simulink library "utility_service_lib"  (Simulink 8.1)
settings: Solver=ode45  StartTime=0.0  StopTime=10.0  RelTol=1e-3
undefined symbols (not defined in the file or in its folder): fdesignblkfcn, gcbh
libraries: rtio_opalrt_common x15, simulink x10, simulink_extras x8, rtio_opalrt_op5142ex1 x6, EasyGen3500_GensetSignalScaling_lib x2, rtlab x1
(part 1 of 2)
settings Model: Creator=RE25624  LastModifiedBy=RE25624

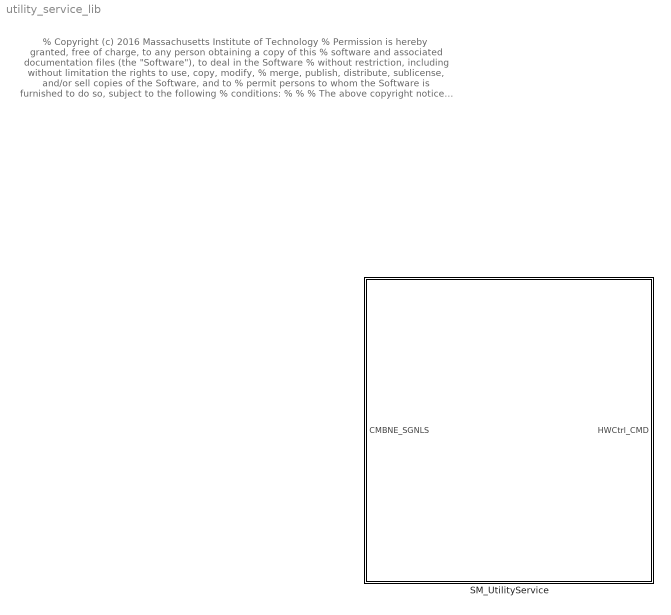
== system utility_service_lib ==
  note: % Copyright (c) 2016 Massachusetts Institute of Technology
      | % Permission is hereby granted, free of charge, to any person obtaining a copy of this
      | % software and associated documentation files (the "Software"), to deal in the Software
      | % without restriction, including without limitation the rights to use, copy, modify,
      | % merge, publish, distribute, sublicense, and/or sell copies of the Software, and to
      | % permit persons to whom the Software is furnished to do so, subject to the following
      | % conditions:
      | %
      | %
      | % The above copyright notice and this permission notice shall be included in
      | % all copies or substantial portions of the Software.
      | %
      | % THE SOFTWARE IS PROVIDED "AS IS", WITHOUT WARRANTY OF ANY KIND, EXPRESS OR IMPLIED,
      | % INCLUDING BUT NOT LIMITED TO THE WARRANTIES OF MERCHANTABILITY, FITNESS FOR A
      | % PARTICULAR PURPOSE AND NONINFRINGEMENT. IN NO EVENT SHALL THE AUTHORS OR COPYRIGHT
      | % HOLDERS BE LIABLE FOR ANY CLAIM, DAMAGES OR OTHER LIABILITY, WHETHER IN AN ACTION
      | % OF CONTRACT, TORT OR OTHERWISE, ARISING FROM, OUT OF OR IN CONNECTION WITH THE
      | % SOFTWARE OR THE USE OR OTHER DEALINGS IN THE SOFTWARE.
      | %
      | %
      | %%
  SM_UtilityService : Subsystem

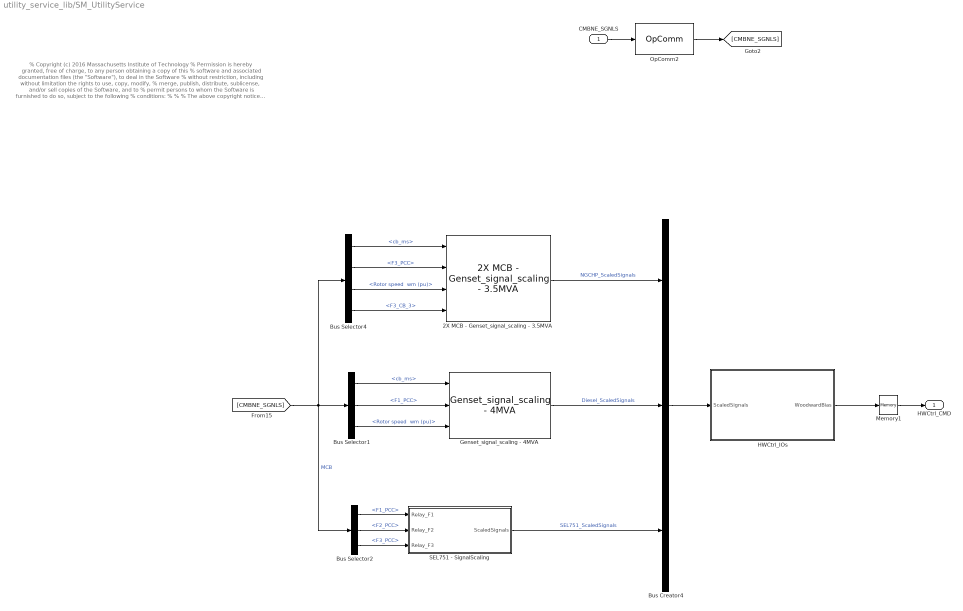
== system utility_service_lib/SM_UtilityService ==
  note: % Copyright (c) 2016 Massachusetts Institute of Technology
      | % Permission is hereby granted, free of charge, to any person obtaining a copy of this
      | % software and associated documentation files (the "Software"), to deal in the Software
      | % without restriction, including without limitation the rights to use, copy, modify,
      | % merge, publish, distribute, sublicense, and/or sell copies of the Software, and to
      | % permit persons to whom the Software is furnished to do so, subject to the following
      | % conditions:
      | %
      | %
      | % The above copyright notice and this permission notice shall be included in
      | % all copies or substantial portions of the Software.
      | %
      | % THE SOFTWARE IS PROVIDED "AS IS", WITHOUT WARRANTY OF ANY KIND, EXPRESS OR IMPLIED,
      | % INCLUDING BUT NOT LIMITED TO THE WARRANTIES OF MERCHANTABILITY, FITNESS FOR A
      | % PARTICULAR PURPOSE AND NONINFRINGEMENT. IN NO EVENT SHALL THE AUTHORS OR COPYRIGHT
      | % HOLDERS BE LIABLE FOR ANY CLAIM, DAMAGES OR OTHER LIABILITY, WHETHER IN AN ACTION
      | % OF CONTRACT, TORT OR OTHERWISE, ARISING FROM, OUT OF OR IN CONNECTION WITH THE
      | % SOFTWARE OR THE USE OR OTHER DEALINGS IN THE SOFTWARE.
      | %
      | %
      | %%
  CMBNE_SGNLS : Inport
  2X MCB - Genset_signal_scaling - 3.5MVA : EasyGen3500_GensetSignalScaling_lib/2X MCB - Genset_signal_scaling - 3.5MVA  Vpk_mcb=11268  watt_mcb=3150000  Vpk_gcb=11268  watt_gcb=3150000  rated_rpm=1800  wm_noise_bias=0.02
  Bus Creator4 : BusCreator  Inputs=3
  Bus Selector1 : BusSelector  OutputSignals="F1_MS_IN.DIESEL_DATA.DIESEL_GCB.cb_ms,F1_MS_IN.CB_DATA.F1_PCC,F1_MS_IN.DIESEL_DATA.Gen2_meas.w.w.Rotor speed  wm (pu)"
  Bus Selector2 : BusSelector  OutputSignals=F1_MS_IN.CB_DATA.F1_PCC,F2_MS_IN.CB_DATA.F2_PCC,F3_MS_IN.CB_DATA.F3_PCC
  Bus Selector4 : BusSelector  OutputSignals="F3_MS_IN.NG_CHP_DATA.NG_CHP_GCB.cb_ms,F3_MS_IN.CB_DATA.F3_PCC,F3_MS_IN.NG_CHP_DATA.Gen1_meas.w.w.Rotor speed  wm (pu),F3_MS_IN.CB_DATA.F3_CB_3"
  Genset_signal_scaling - 4MVA : EasyGen3500_GensetSignalScaling_lib/Genset_signal_scaling - 4MVA  Vpk_mcb=11268  watt_mcb=3600000  Vpk_gcb=11268  watt_gcb=3600000  rated_rpm=1800  wm_noise_bias=0.02
  HWCtrl_IOs : Subsystem
  Memory1 : Memory
  OpComm2 : rtlab/OpComm  nbport=1  groupe_acq=1  subsys_rate=0  st=0  Synchronization=on  Interpolation=on  Threshold=1.0  Missed_Data=off  Sim_Time=off  Samples=off  dynSigOut=off  from_console=0  warning_done=off  writeOpCommFile=off  Offset=off
  SEL751 - SignalScaling : Subsystem  mask(SEL751 - SignalScaling){ct_ratio=1/1250, pt_ratio=1/1800}
      mask prompts: ct_ratio "CT Ratio"; pt_ratio "PT Ratio"
      mask help: CT and PT ratios should match the settings in the corresponding SEL751
  HWCtrl_CMD : Outport
  wires:
  Bus Selector4/4 -> 2X MCB - Genset_signal_scaling - 3.5MVA/4  "<F3_CB_3>"
  Bus Selector2/3 -> SEL751 - SignalScaling/3(Relay_F3)  "<F3_PCC>"
  Bus Selector2/1 -> SEL751 - SignalScaling/1(Relay_F1)  "<F1_PCC>"
  Bus Selector2/2 -> SEL751 - SignalScaling/2(Relay_F2)  "<F2_PCC>"
  SEL751 - SignalScaling/1(ScaledSignals) -> Bus Creator4/3  "SEL751_ScaledSignals"
  OpComm2/1 -> [CMBNE_SGNLS]
  CMBNE_SGNLS/1 -> OpComm2/1
  Bus Selector1/1 -> Genset_signal_scaling - 4MVA/1  "<cb_ms>"
  Bus Selector1/2 -> Genset_signal_scaling - 4MVA/2  "<F1_PCC>"
  Bus Selector1/3 -> Genset_signal_scaling - 4MVA/3  "<Rotor speed  wm (pu)>"
  HWCtrl_IOs/1(WoodwardBias) -> Memory1/1
  Bus Creator4/1 -> HWCtrl_IOs/1(ScaledSignals)
  Bus Selector4/1 -> 2X MCB - Genset_signal_scaling - 3.5MVA/1  "<cb_ms>"
  Bus Selector4/2 -> 2X MCB - Genset_signal_scaling - 3.5MVA/2  "<F3_PCC>"
  Bus Selector4/3 -> 2X MCB - Genset_signal_scaling - 3.5MVA/3  "<Rotor speed  wm (pu)>"
  [CMBNE_SGNLS] -> Bus Selector1/1, Bus Selector2/1, Bus Selector4/1  "MCB"
  Genset_signal_scaling - 4MVA/1 -> Bus Creator4/2  "Diesel_ScaledSignals"
  2X MCB - Genset_signal_scaling - 3.5MVA/1 -> Bus Creator4/1  "NGCHP_ScaledSignals"
  Memory1/1 -> HWCtrl_CMD/1

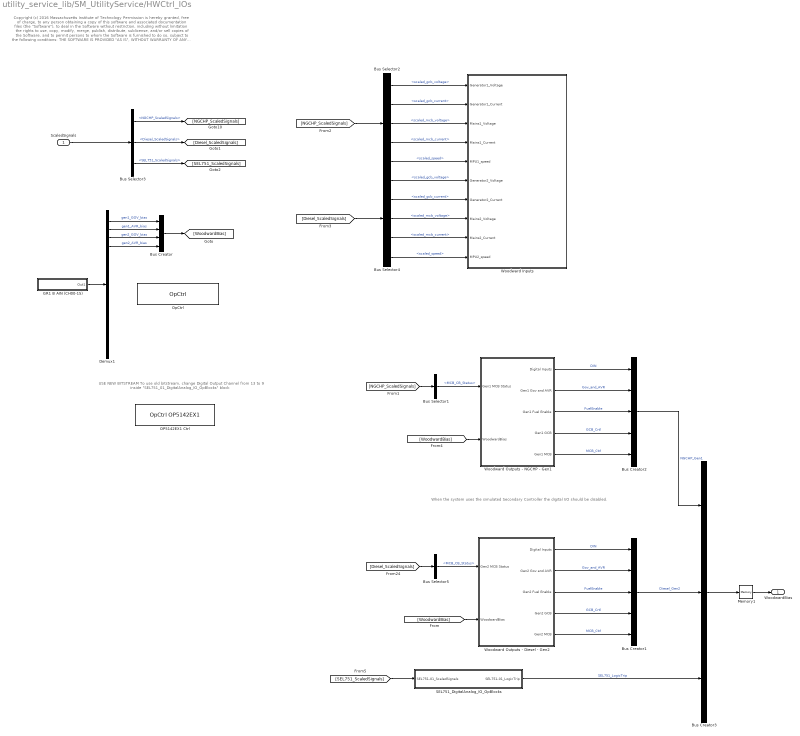
== system utility_service_lib/SM_UtilityService/HWCtrl_IOs ==
  note: USE NEW  BITSTREAM
      | To use old bitstream, change Digital Output Channel from 13 to 9 inside
      | "SEL751_01_DigitalAnalog_IO_OpBlocks" block
  note: Copyright (c) 2016 Massachusetts Institute of Technology
      | Permission is hereby granted, free of charge, to any person obtaining a copy of this software and associated documentation files (the "Software"), to deal
      | in the Software without restriction, including without limitation the rights to use, copy, modify, merge, publish, distribute, sublicense, and/or sell copies of the
      | Software, and to permit persons to whom the Software is furnished to do so, subject to the following conditions:
      |
      | THE SOFTWARE IS PROVIDED "AS IS", WITHOUT WARRANTY OF ANY KIND, EXPRESS OR IMPLIED, INCLUDING BUT NOT LIMITED TO THE
      | WARRANTIES OF MERCHANTABILITY, FITNESS FOR A PARTICULAR PURPOSE AND NONINFRINGEMENT. IN NO EVENT SHALL THE AUTHORS
      | OR COPYRIGHT HOLDERS BE LIABLE FOR ANY CLAIM, DAMAGES OR OTHER LIABILITY, WHETHER IN AN ACTION OF CONTRACT, TORT OR
      | OTHERWISE, ARISING FROM, OUT OF OR IN CONNECTION WITH THE SOFTWARE OR THE USE OR OTHER DEALINGS IN THE SOFTWARE
  note: When the system uses the simulated
      | Secondary Controller the digital I/O
      | should be disabled.
  ScaledSignals : Inport
  Bus Creator : BusCreator
  Bus Creator1 : BusCreator  Inputs=5
  Bus Creator2 : BusCreator  Inputs=5
  Bus Creator3 : BusCreator  Inputs=3
  Bus Selector1 : BusSelector  OutputSignals=MCB_CB_Status
  Bus Selector2 : BusSelector  OutputSignals=scaled_gcb_voltage,scaled_gcb_current,scaled_mcb_voltage,scaled_mcb_current,scaled_speed
  Bus Selector3 : BusSelector  OutputSignals=NGCHP_ScaledSignals,Diesel_ScaledSignals,SEL751_ScaledSignals
  Bus Selector4 : BusSelector  OutputSignals=scaled_gcb_voltage,scaled_gcb_current,scaled_mcb_voltage,scaled_mcb_current,scaled_speed
  Bus Selector5 : BusSelector  OutputSignals=MCB_CB_Status
  Demux1 : Demux  Outputs=16
  GR1 B AIN (CH00-15) : Subsystem
  Memory1 : Memory
  OP5142EX1 Ctrl : rtio_opalrt_op5142ex1/OpCtrl OP5142EX1  CtrlName='OP5142EX1 Ctrl'  boardid=1  BitstreamFilename=OP5142_1-EX-0000-2_3_4_54-16AIO_48AO_32DO_16DIO_16selDIO_CD-FF-01.bin  numconfig=-1  mode=Slave  externalClock=off  decimRtsi=0  calibIO=off  SampleTime=0  loadinport=-1
  OpCtrl : rtio_opalrt_common/OpCtrl  CtrlName='OpCtrl'  boardid=0  BitstreamFilename=VC707_2-EX-0001-2_3_2_20-48AIO16DIO16DIOSel-02-01.bin  numconfig=-1  mode=Master  externalClock=off  decimRtsi=0  calibIO=off  SampleTime=0  loadinport=-1  BoardType=VC707  SecondaryPresent=off  sync_type=Audio
  SEL751_DigitalAnalog_IO_OpBlocks : Subsystem
  Woodward Inputs : Subsystem
  Woodward Outputs - Diesel - Gen2 : Subsystem
  Woodward Outputs - NGCHP - Gen1 : Subsystem
  WoodwardBias : Outport
  wires:
  [SEL751_ScaledSignals] -> SEL751_DigitalAnalog_IO_OpBlocks/1(SEL751-01_ScaledSignals)
  Bus Selector3/3 -> [SEL751_ScaledSignals]  "<SEL751_ScaledSignals>"
  SEL751_DigitalAnalog_IO_OpBlocks/1(SEL751-01_LogicTrip) -> Bus Creator3/3  "SEL751_LogicTrip"
  ScaledSignals/1 -> Bus Selector3/1
  Bus Selector3/1 -> [NGCHP_ScaledSignals]  "<NGCHP_ScaledSignals>"
  Bus Selector3/2 -> [Diesel_ScaledSignals]  "<Diesel_ScaledSignals>"
  [NGCHP_ScaledSignals] -> Bus Selector2/1
  Bus Selector2/5 -> Woodward Inputs/5(MPU1_speed)  "<scaled_speed>"
  Bus Selector2/4 -> Woodward Inputs/4(Mains1_Current)  "<scaled_mcb_current>"
  Bus Selector2/3 -> Woodward Inputs/3(Mains1_Voltage)  "<scaled_mcb_voltage>"
  Bus Selector2/2 -> Woodward Inputs/2(Generator1_Current)  "<scaled_gcb_current>"
  Bus Selector2/1 -> Woodward Inputs/1(Generator1_Voltage)  "<scaled_gcb_voltage>"
  [Diesel_ScaledSignals] -> Bus Selector4/1
  Bus Selector4/1 -> Woodward Inputs/6(Generator2_Voltage)  "<scaled_gcb_voltage>"
  Bus Selector4/2 -> Woodward Inputs/7(Generator2_Current)  "<scaled_gcb_current>"
  Bus Selector4/3 -> Woodward Inputs/8(Mains2_Voltage)  "<scaled_mcb_voltage>"
  Bus Selector4/4 -> Woodward Inputs/9(Mains2_Current)  "<scaled_mcb_current>"
  Bus Selector4/5 -> Woodward Inputs/10(MPU2_speed)  "<scaled_speed>"
  GR1 B AIN (CH00-15)/1(Out1) -> Demux1/1
  Demux1/1 -> Bus Creator/1  "gen1_GOV_bias"
  Demux1/2 -> Bus Creator/2  "gen1_AVR_bias"
  Demux1/3 -> Bus Creator/3  "gen2_GOV_bias"
  Demux1/4 -> Bus Creator/4  "gen2_AVR_bias"
  Bus Selector5/1 -> Woodward Outputs - Diesel - Gen2/1(Gen2 MCB Status)  "<MCB_CB_Status>"
  [WoodwardBias] -> Woodward Outputs - Diesel - Gen2/2(WoodwardBias)
  [Diesel_ScaledSignals] -> Bus Selector5/1
  Woodward Outputs - Diesel - Gen2/2(Gen2 Gov and AVR) -> Bus Creator1/2  "Gov_and_AVR"
  Woodward Outputs - Diesel - Gen2/3(Gen2 Fuel Enable) -> Bus Creator1/3  "FuelEnable"
  Woodward Outputs - Diesel - Gen2/4(Gen2 GCB) -> Bus Creator1/4  "GCB_Crtl"
  Woodward Outputs - Diesel - Gen2/5(Gen2 MCB) -> Bus Creator1/5  "MCB_Ctrl"
  Bus Creator1/1 -> Bus Creator3/2  "Diesel_Gen2"
  Bus Creator3/1 -> Memory1/1
  Bus Creator2/1 -> Bus Creator3/1  "NGCHP_Gen1"
  Woodward Outputs - NGCHP - Gen1/1(Digital Inputs) -> Bus Creator2/1  "DIN"
  Woodward Outputs - NGCHP - Gen1/2(Gen1 Gov and AVR) -> Bus Creator2/2  "Gov_and_AVR"
  Woodward Outputs - NGCHP - Gen1/3(Gen1 Fuel Enable) -> Bus Creator2/3  "FuelEnable"
  Woodward Outputs - NGCHP - Gen1/4(Gen1 GCB) -> Bus Creator2/4  "GCB_Crtl"
  Woodward Outputs - Diesel - Gen2/1(Digital Inputs) -> Bus Creator1/1  "DIN"
  Woodward Outputs - NGCHP - Gen1/5(Gen1 MCB) -> Bus Creator2/5  "MCB_Ctrl"
  [WoodwardBias] -> Woodward Outputs - NGCHP - Gen1/2(WoodwardBias)
  [NGCHP_ScaledSignals] -> Bus Selector1/1
  Bus Selector1/1 -> Woodward Outputs - NGCHP - Gen1/1(Gen1 MCB Status)  "<MCB_CB_Status>"
  Memory1/1 -> WoodwardBias/1
  Bus Creator/1 -> [WoodwardBias]

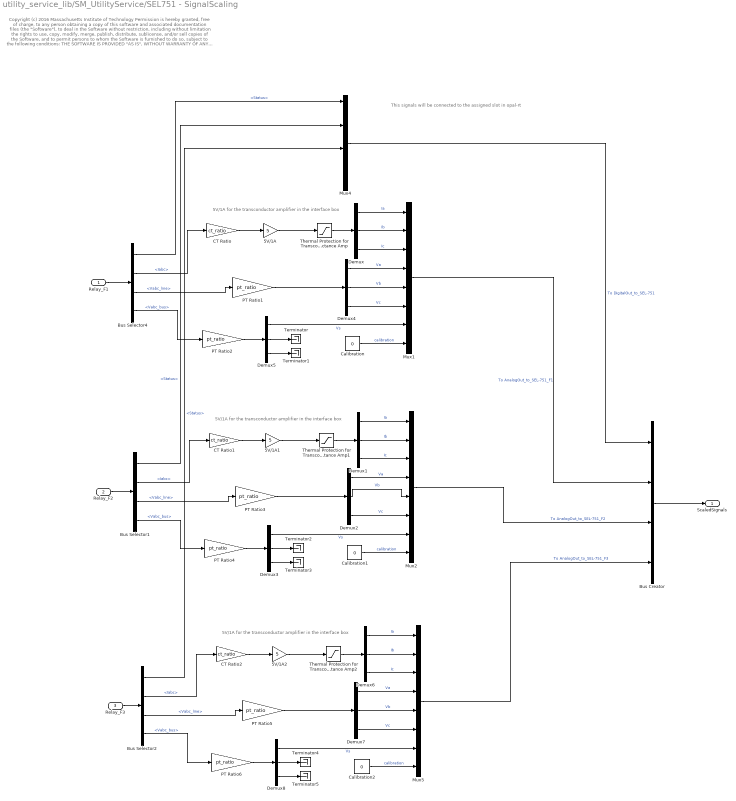
== system utility_service_lib/SM_UtilityService/SEL751 - SignalScaling ==
  note: Copyright (c) 2016 Massachusetts Institute of Technology
      | Permission is hereby granted, free of charge, to any person obtaining a copy of this software and associated documentation files (the "Software"), to deal
      | in the Software without restriction, including without limitation the rights to use, copy, modify, merge, publish, distribute, sublicense, and/or sell copies of the
      | Software, and to permit persons to whom the Software is furnished to do so, subject to the following conditions:
      |
      | THE SOFTWARE IS PROVIDED "AS IS", WITHOUT WARRANTY OF ANY KIND, EXPRESS OR IMPLIED, INCLUDING BUT NOT LIMITED TO THE
      | WARRANTIES OF MERCHANTABILITY, FITNESS FOR A PARTICULAR PURPOSE AND NONINFRINGEMENT. IN NO EVENT SHALL THE AUTHORS
      | OR COPYRIGHT HOLDERS BE LIABLE FOR ANY CLAIM, DAMAGES OR OTHER LIABILITY, WHETHER IN AN ACTION OF CONTRACT, TORT OR
      | OTHERWISE, ARISING FROM, OUT OF OR IN CONNECTION WITH THE SOFTWARE OR THE USE OR OTHER DEALINGS IN THE SOFTWARE
  note: This signals will be connected to the assigned slot in opal-rt
  note: 5V/1A for the transconductor
      | amplifier in the interface box
  note: 5V/1A for the transconductor
      | amplifier in the interface box
  note: 5V/1A for the transconductor
      | amplifier in the interface box
  Relay_F1 : Inport
  Relay_F2 : Inport  Port=2
  Relay_F3 : Inport  Port=3
  5V/1A : Gain  Gain=5
  5V/1A1 : Gain  Gain=5
  5V/1A2 : Gain  Gain=5
  Bus Creator : BusCreator
  Bus Selector1 : BusSelector  OutputSignals=Status,Iabc,Vabc_line,Vabc_bus
  Bus Selector2 : BusSelector  OutputSignals=Status,Iabc,Vabc_line,Vabc_bus
  Bus Selector4 : BusSelector  OutputSignals=Status,Iabc,Vabc_line,Vabc_bus
  CT Ratio : Gain  Gain=ct_ratio
  CT Ratio1 : Gain  Gain=ct_ratio
  CT Ratio2 : Gain  Gain=ct_ratio
  Calibration : Constant  Value=0
  Calibration1 : Constant  Value=0
  Calibration2 : Constant  Value=0
  Demux{,1..8} (9 alike) : Demux  Outputs=3
  Mux{1..2,4..5} (4 alike) : Mux  Inputs=8
  PT Ratio{1..6} (6 alike) : Gain  Gain=pt_ratio
  Terminator{,1..5} (6 alike) : Terminator
  Thermal Protection for Transconductance Amp : Saturate  UpperLimit=5  LowerLimit=-5
  Thermal Protection for Transconductance Amp1 : Saturate  UpperLimit=5  LowerLimit=-5
  Thermal Protection for Transconductance Amp2 : Saturate  UpperLimit=5  LowerLimit=-5
  ScaledSignals : Outport
  wires:
  5V/1A/1 -> Thermal Protection for Transconductance Amp/1
  Bus Creator/1 -> ScaledSignals/1
  Demux5/3 -> Terminator1/1
  Demux5/2 -> Terminator/1
  Thermal Protection for Transconductance Amp/1 -> Demux/1
  PT Ratio2/1 -> Demux5/1
  PT Ratio1/1 -> Demux4/1
  CT Ratio/1 -> 5V/1A/1
  Relay_F1/1 -> Bus Selector4/1
  Demux/2 -> Mux1/2  "Ib"
  Demux/3 -> Mux1/3  "Ic"
  Demux/1 -> Mux1/1  "Ia"
  Mux1/1 -> Bus Creator/2  "To AnalogOut_to_SEL-751_F1"
  Mux4/1 -> Bus Creator/1  "To DigitalOut_to_SEL-751"
  Bus Selector4/1 -> Mux4/1  "<Status>"
  Calibration/1 -> Mux1/8  "calibration"
  Bus Selector4/3 -> PT Ratio1/1  "<Vabc_line>"
  Demux5/1 -> Mux1/7  "Vs"
  Bus Selector4/4 -> PT Ratio2/1  "<Vabc_bus>"
  Demux4/3 -> Mux1/6  "Vc"
  Demux4/2 -> Mux1/5  "Vb"
  Demux4/1 -> Mux1/4  "Va"
  Bus Selector4/2 -> CT Ratio/1  "<Iabc>"
  5V/1A1/1 -> Thermal Protection for Transconductance Amp1/1
  Demux3/3 -> Terminator3/1
  Demux3/2 -> Terminator2/1
  Thermal Protection for Transconductance Amp1/1 -> Demux1/1
  PT Ratio4/1 -> Demux3/1
  PT Ratio3/1 -> Demux2/1
  CT Ratio1/1 -> 5V/1A1/1
  Demux1/2 -> Mux2/2  "Ib"
  Demux1/3 -> Mux2/3  "Ic"
  Demux1/1 -> Mux2/1  "Ia"
  Mux2/1 -> Bus Creator/3  "To AnalogOut_to_SEL-751_F2"
  Bus Selector1/1 -> Mux4/3  "<Status>"
  Calibration1/1 -> Mux2/8  "calibration"
  Bus Selector1/3 -> PT Ratio3/1  "<Vabc_line>"
  Demux3/1 -> Mux2/7  "Vs"
  Bus Selector1/4 -> PT Ratio4/1  "<Vabc_bus>"
  Demux2/3 -> Mux2/6  "Vc"
  Demux2/2 -> Mux2/5  "Vb"
  Demux2/1 -> Mux2/4  "Va"
  Bus Selector1/2 -> CT Ratio1/1  "<Iabc>"
  5V/1A2/1 -> Thermal Protection for Transconductance Amp2/1
  Demux8/3 -> Terminator5/1
  Demux8/2 -> Terminator4/1
  Thermal Protection for Transconductance Amp2/1 -> Demux6/1
  PT Ratio6/1 -> Demux8/1
  PT Ratio5/1 -> Demux7/1
  CT Ratio2/1 -> 5V/1A2/1
  Demux6/2 -> Mux5/2  "Ib"
  Demux6/3 -> Mux5/3  "Ic"
  Demux6/1 -> Mux5/1  "Ia"
  Mux5/1 -> Bus Creator/4  "To AnalogOut_to_SEL-751_F3"
  Bus Selector2/1 -> Mux4/5  "<Status>"
  Calibration2/1 -> Mux5/8  "calibration"
  Bus Selector2/3 -> PT Ratio5/1  "<Vabc_line>"
  Demux8/1 -> Mux5/7  "Vs"
  Bus Selector2/4 -> PT Ratio6/1  "<Vabc_bus>"
  Demux7/3 -> Mux5/6  "Vc"
  Demux7/2 -> Mux5/5  "Vb"
  Demux7/1 -> Mux5/4  "Va"
  Bus Selector2/2 -> CT Ratio2/1  "<Iabc>"
  Relay_F2/1 -> Bus Selector1/1
  Relay_F3/1 -> Bus Selector2/1

== system utility_service_lib/SM_UtilityService/HWCtrl_IOs/GR1 B AIN (CH00-15) ==
  AnalogIn : rtio_opalrt_common/AnalogIn  CtrlName='OpCtrl'  portNb=1  FcnNos=Slot 1 Module B Subsection 1  size=16  maxcount=8  count=8  numchan=8  sampleTime=0
      settings: AttributesFormatString=%<CtrlName>
  AnalogIn1 : rtio_opalrt_common/AnalogIn  CtrlName='OpCtrl'  portNb=2  FcnNos=Slot 1 Module B Subsection 2  size=16  maxcount=8  count=8  numchan=8  sampleTime=0
      settings: AttributesFormatString=%<CtrlName>
  Mux6 : Mux  Inputs=2
  Terminator2 : Terminator
  Terminator3 : Terminator
  Out1 : Outport
  wires:
  AnalogIn/1 -> Mux6/1
  AnalogIn1/1 -> Mux6/2
  AnalogIn/2 -> Terminator2/1
  AnalogIn1/2 -> Terminator3/1
  Mux6/1 -> Out1/1

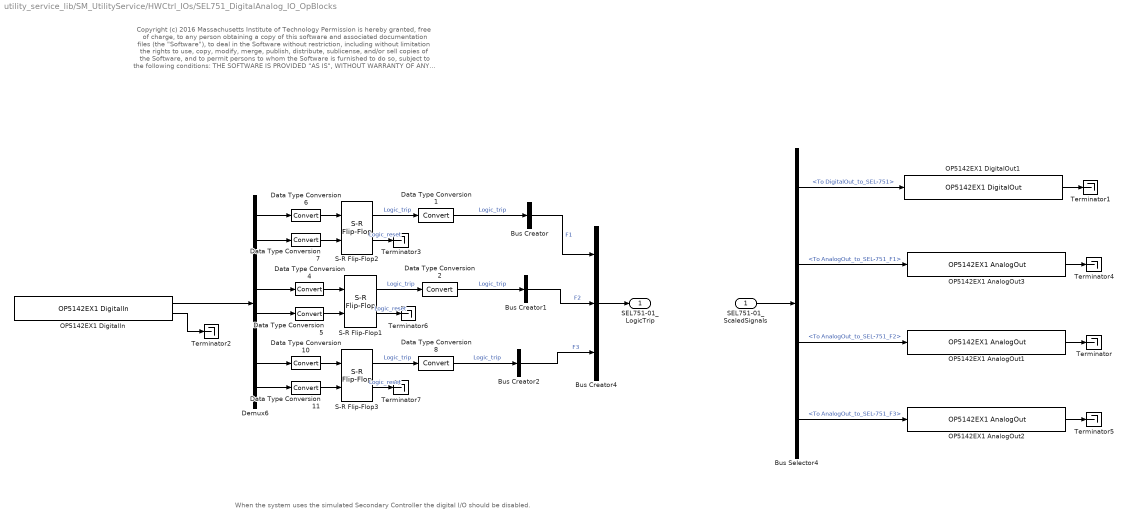
== system utility_service_lib/SM_UtilityService/HWCtrl_IOs/SEL751_DigitalAnalog_IO_OpBlocks ==
  note: Copyright (c) 2016 Massachusetts Institute of Technology
      | Permission is hereby granted, free of charge, to any person obtaining a copy of this software and associated documentation files (the "Software"), to deal
      | in the Software without restriction, including without limitation the rights to use, copy, modify, merge, publish, distribute, sublicense, and/or sell copies of the
      | Software, and to permit persons to whom the Software is furnished to do so, subject to the following conditions:
      |
      | THE SOFTWARE IS PROVIDED "AS IS", WITHOUT WARRANTY OF ANY KIND, EXPRESS OR IMPLIED, INCLUDING BUT NOT LIMITED TO THE
      | WARRANTIES OF MERCHANTABILITY, FITNESS FOR A PARTICULAR PURPOSE AND NONINFRINGEMENT. IN NO EVENT SHALL THE AUTHORS
      | OR COPYRIGHT HOLDERS BE LIABLE FOR ANY CLAIM, DAMAGES OR OTHER LIABILITY, WHETHER IN AN ACTION OF CONTRACT, TORT OR
      | OTHERWISE, ARISING FROM, OUT OF OR IN CONNECTION WITH THE SOFTWARE OR THE USE OR OTHER DEALINGS IN THE SOFTWARE
  note: When the system uses the simulated
      | Secondary Controller the digital I/O
      | should be disabled.
  SEL751-01_ScaledSignals : Inport
  Bus Creator : BusCreator  Inputs=1
  Bus Creator1 : BusCreator  Inputs=1
  Bus Creator2 : BusCreator  Inputs=1
  Bus Creator4 : BusCreator  Inputs=3
  Bus Selector4 : BusSelector  OutputSignals=To DigitalOut_to_SEL-751,To AnalogOut_to_SEL-751_F1,To AnalogOut_to_SEL-751_F2,To AnalogOut_to_SEL-751_F3
  Data Type Conversion{1..2,4..8,10..11} (9 alike) : DataTypeConversion
  Demux6 : Demux  Outputs=8
  OP5142EX1 AnalogOut1 : rtio_opalrt_op5142ex1/OP5142EX1 AnalogOut  CtrlName='OP5142EX1 Ctrl'  portNb=2  FcnNos=Slot 1 Module A Subsection 2  size=16  maxcount=8  count=8  numchan=8  israngeinput=off  voltagerange=[-16 ... 16]  slot=0  side=0  mismatch=0  slotside=Slot_1_Module_A
      settings: AttributesFormatString=%<CtrlName>
  OP5142EX1 AnalogOut2 : rtio_opalrt_op5142ex1/OP5142EX1 AnalogOut  CtrlName='OP5142EX1 Ctrl'  portNb=3  FcnNos=Slot 2 Module A Subsection 1  size=16  maxcount=8  count=8  numchan=8  israngeinput=off  voltagerange=[-16 ... 16]  slot=1  side=0  mismatch=0  slotside=Slot_2_Module_A
      settings: AttributesFormatString=%<CtrlName>
  OP5142EX1 AnalogOut3 : rtio_opalrt_op5142ex1/OP5142EX1 AnalogOut  CtrlName='OP5142EX1 Ctrl'  portNb=1  FcnNos=Slot 1 Module A Subsection 1  size=16  maxcount=8  count=8  numchan=8  israngeinput=off  voltagerange=[-16 ... 16]  slot=0  side=0  mismatch=0  slotside=Slot_1_Module_A
      settings: AttributesFormatString=%<CtrlName>
  OP5142EX1 DigitalIn : rtio_opalrt_op5142ex1/OP5142EX1 DigitalIn  CtrlName='OP5142EX1 Ctrl'  portNb=3  FcnNos=Slot 4 Module A Subsection 1  size=1  maxcount=8  count=8  sampleTime=0  numchan=8
      settings: AttributesFormatString=%<CtrlName>
  OP5142EX1 DigitalOut1 : rtio_opalrt_op5142ex1/OP5142EX1 DigitalOut  CtrlName='OP5142EX1 Ctrl'  portNb=13  FcnNos=Slot 4 Module B Subsection 1  size=1  maxcount=8  count=8  numchan=8
      settings: AttributesFormatString=%<CtrlName>
  S-R Flip-Flop1 : simulink_extras/Flip Flops/S-R Flip-Flop  initial_condition=1
  S-R Flip-Flop2 : simulink_extras/Flip Flops/S-R Flip-Flop  initial_condition=1
  S-R Flip-Flop3 : simulink_extras/Flip Flops/S-R Flip-Flop  initial_condition=1
  Terminator{,1..7} (8 alike) : Terminator
  SEL751-01_LogicTrip : Outport
  wires:
  Bus Selector4/2 -> OP5142EX1 AnalogOut3/1  "<To AnalogOut_to_SEL-751_F1>"
  Bus Selector4/3 -> OP5142EX1 AnalogOut1/1  "<To AnalogOut_to_SEL-751_F2>"
  Bus Selector4/4 -> OP5142EX1 AnalogOut2/1  "<To AnalogOut_to_SEL-751_F3>"
  S-R Flip-Flop2/2 -> Terminator3/1  "Logic_reset"
  S-R Flip-Flop1/2 -> Terminator6/1  "Logic_reset"
  S-R Flip-Flop3/2 -> Terminator7/1  "Logic_reset"
  Demux6/1 -> Data Type Conversion6/1
  Demux6/2 -> Data Type Conversion7/1
  Demux6/8 -> Data Type Conversion11/1
  Demux6/7 -> Data Type Conversion10/1
  S-R Flip-Flop3/1 -> Data Type Conversion8/1  "Logic_trip"
  Data Type Conversion10/1 -> S-R Flip-Flop3/1
  Data Type Conversion11/1 -> S-R Flip-Flop3/2
  S-R Flip-Flop2/1 -> Data Type Conversion1/1  "Logic_trip"
  Data Type Conversion6/1 -> S-R Flip-Flop2/1
  Data Type Conversion7/1 -> S-R Flip-Flop2/2
  S-R Flip-Flop1/1 -> Data Type Conversion2/1  "Logic_trip"
  OP5142EX1 DigitalIn/2 -> Terminator2/1
  OP5142EX1 DigitalIn/1 -> Demux6/1
  Data Type Conversion4/1 -> S-R Flip-Flop1/1
  Data Type Conversion5/1 -> S-R Flip-Flop1/2
  Demux6/4 -> Data Type Conversion4/1
  Demux6/5 -> Data Type Conversion5/1
  OP5142EX1 AnalogOut3/1 -> Terminator4/1
  OP5142EX1 AnalogOut2/1 -> Terminator5/1
  SEL751-01_ScaledSignals/1 -> Bus Selector4/1
  Bus Selector4/1 -> OP5142EX1 DigitalOut1/1  "<To DigitalOut_to_SEL-751>"
  OP5142EX1 AnalogOut1/1 -> Terminator/1
  OP5142EX1 DigitalOut1/1 -> Terminator1/1
  Bus Creator1/1 -> Bus Creator4/2  "F2"
  Bus Creator2/1 -> Bus Creator4/3  "F3"
  Bus Creator/1 -> Bus Creator4/1  "F1"
  Data Type Conversion8/1 -> Bus Creator2/1  "Logic_trip"
  Data Type Conversion2/1 -> Bus Creator1/1  "Logic_trip"
  Bus Creator4/1 -> SEL751-01_LogicTrip/1
  Data Type Conversion1/1 -> Bus Creator/1  "Logic_trip"

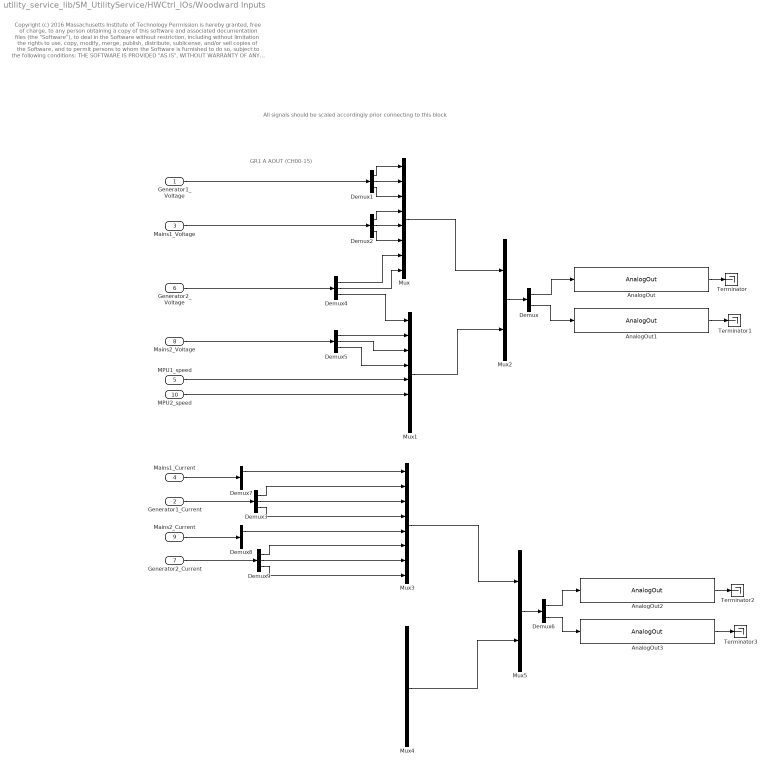
== system utility_service_lib/SM_UtilityService/HWCtrl_IOs/Woodward Inputs ==
  note: All signals should be scaled accordingly prior connecting to this block
  note: GR1 A AOUT (CH00-15)
  note: Copyright (c) 2016 Massachusetts Institute of Technology
      | Permission is hereby granted, free of charge, to any person obtaining a copy of this software and associated documentation files (the "Software"), to deal
      | in the Software without restriction, including without limitation the rights to use, copy, modify, merge, publish, distribute, sublicense, and/or sell copies of the
      | Software, and to permit persons to whom the Software is furnished to do so, subject to the following conditions:
      |
      | THE SOFTWARE IS PROVIDED "AS IS", WITHOUT WARRANTY OF ANY KIND, EXPRESS OR IMPLIED, INCLUDING BUT NOT LIMITED TO THE
      | WARRANTIES OF MERCHANTABILITY, FITNESS FOR A PARTICULAR PURPOSE AND NONINFRINGEMENT. IN NO EVENT SHALL THE AUTHORS
      | OR COPYRIGHT HOLDERS BE LIABLE FOR ANY CLAIM, DAMAGES OR OTHER LIABILITY, WHETHER IN AN ACTION OF CONTRACT, TORT OR
      | OTHERWISE, ARISING FROM, OUT OF OR IN CONNECTION WITH THE SOFTWARE OR THE USE OR OTHER DEALINGS IN THE SOFTWARE
  Generator1_Voltage : Inport
  Generator1_Current : Inport  Port=2
  Mains1_Voltage : Inport  Port=3
  Mains1_Current : Inport  Port=4
  MPU1_speed : Inport  Port=5
  Generator2_Voltage : Inport  Port=6
  Generator2_Current : Inport  Port=7
  Mains2_Voltage : Inport  Port=8
  Mains2_Current : Inport  Port=9
  MPU2_speed : Inport  Port=10
  AnalogOut : rtio_opalrt_common/AnalogOut  CtrlName='OpCtrl'  portNb=1  FcnNos=Slot 1 Module A Subsection 1  size=16  maxcount=8  count=8  numchan=8  israngeinput=off  voltagerange=[-16 ... 16]  slot=0  side=0  mismatch=0  slotside=Slot_1_Module_A
      settings: AttributesFormatString=%<CtrlName>
  AnalogOut1 : rtio_opalrt_common/AnalogOut  CtrlName='OpCtrl'  portNb=2  FcnNos=Slot 1 Module A Subsection 2  size=16  maxcount=8  count=8  numchan=8  israngeinput=off  voltagerange=[-16 ... 16]  slot=0  side=0  mismatch=0  slotside=Slot_1_Module_A
      settings: AttributesFormatString=%<CtrlName>
  AnalogOut2 : rtio_opalrt_common/AnalogOut  CtrlName='OpCtrl'  portNb=3  FcnNos=Slot 2 Module A Subsection 1  size=16  maxcount=8  count=8  numchan=8  israngeinput=off  voltagerange=[-16 ... 16]  slot=1  side=0  mismatch=0  slotside=Slot_2_Module_A
      settings: AttributesFormatString=%<CtrlName>
  AnalogOut3 : rtio_opalrt_common/AnalogOut  CtrlName='OpCtrl'  portNb=4  FcnNos=Slot 2 Module A Subsection 2  size=16  maxcount=8  count=8  numchan=8  israngeinput=off  voltagerange=[-16 ... 16]  slot=1  side=0  mismatch=0  slotside=Slot_2_Module_A
      settings: AttributesFormatString=%<CtrlName>
  Demux : Demux  Outputs=2
  Demux{1..5,7..9} (8 alike) : Demux  Outputs=3
  Demux6 : Demux  Outputs=2
  Mux{,1,3..4} (4 alike) : Mux  Inputs=8
  Mux2 : Mux  Inputs=2
  Mux5 : Mux  Inputs=2
  Terminator{,1..3} (4 alike) : Terminator
  wires:
  Demux9/3 -> Mux3/8
  Demux9/2 -> Mux3/7
  Demux9/1 -> Mux3/6
  Generator2_Current/1 -> Demux9/1
  Demux8/1 -> Mux3/5
  Mains2_Current/1 -> Demux8/1
  MPU2_speed/1 -> Mux1/6
  Generator2_Voltage/1 -> Demux4/1
  Mains2_Voltage/1 -> Demux5/1
  Demux7/1 -> Mux3/1
  Mains1_Current/1 -> Demux7/1
  Demux3/3 -> Mux3/4
  Demux3/2 -> Mux3/3
  Demux3/1 -> Mux3/2
  Generator1_Current/1 -> Demux3/1
  AnalogOut2/1 -> Terminator2/1
  AnalogOut3/1 -> Terminator3/1
  Demux6/1 -> AnalogOut2/1
  Demux6/2 -> AnalogOut3/1
  Mux3/1 -> Mux5/1
  Mux4/1 -> Mux5/2
  Mux5/1 -> Demux6/1
  Demux5/3 -> Mux1/4
  Demux5/2 -> Mux1/3
  Demux5/1 -> Mux1/2
  Demux4/3 -> Mux1/1
  Demux4/2 -> Mux/8
  Demux4/1 -> Mux/7
  MPU1_speed/1 -> Mux1/5
  Demux2/3 -> Mux/6
  Demux2/2 -> Mux/5
  Demux2/1 -> Mux/4
  Demux1/3 -> Mux/3
  Demux1/2 -> Mux/2
  Demux1/1 -> Mux/1
  AnalogOut/1 -> Terminator/1
  AnalogOut1/1 -> Terminator1/1
  Demux/1 -> AnalogOut/1
  Demux/2 -> AnalogOut1/1
  Mux/1 -> Mux2/1
  Mux1/1 -> Mux2/2
  Mux2/1 -> Demux/1
  Generator1_Voltage/1 -> Demux1/1
  Mains1_Voltage/1 -> Demux2/1

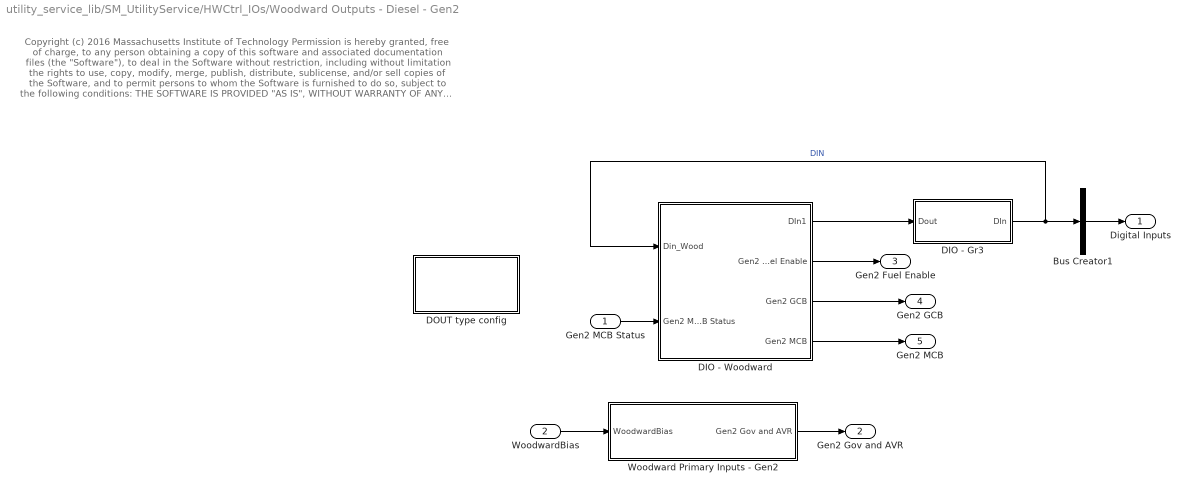
== system utility_service_lib/SM_UtilityService/HWCtrl_IOs/Woodward Outputs - Diesel - Gen2 ==
  note: Copyright (c) 2016 Massachusetts Institute of Technology
      | Permission is hereby granted, free of charge, to any person obtaining a copy of this software and associated documentation files (the "Software"), to deal
      | in the Software without restriction, including without limitation the rights to use, copy, modify, merge, publish, distribute, sublicense, and/or sell copies of the
      | Software, and to permit persons to whom the Software is furnished to do so, subject to the following conditions:
      |
      | THE SOFTWARE IS PROVIDED "AS IS", WITHOUT WARRANTY OF ANY KIND, EXPRESS OR IMPLIED, INCLUDING BUT NOT LIMITED TO THE
      | WARRANTIES OF MERCHANTABILITY, FITNESS FOR A PARTICULAR PURPOSE AND NONINFRINGEMENT. IN NO EVENT SHALL THE AUTHORS
      | OR COPYRIGHT HOLDERS BE LIABLE FOR ANY CLAIM, DAMAGES OR OTHER LIABILITY, WHETHER IN AN ACTION OF CONTRACT, TORT OR
      | OTHERWISE, ARISING FROM, OUT OF OR IN CONNECTION WITH THE SOFTWARE OR THE USE OR OTHER DEALINGS IN THE SOFTWARE
  Gen2 MCB Status : Inport
  WoodwardBias : Inport  Port=2
  Bus Creator1 : BusCreator  Inputs=1
  DIO - Gr3 : Subsystem
  DIO - Woodward : Subsystem
  DOUT type config : Subsystem
  Woodward Primary Inputs - Gen2 : Subsystem
  Digital Inputs : Outport
  Gen2 Gov and AVR : Outport  Port=2
  Gen2 Fuel Enable : Outport  Port=3
  Gen2 GCB : Outport  Port=4
  Gen2 MCB : Outport  Port=5
  wires:
  WoodwardBias/1 -> Woodward Primary Inputs - Gen2/1(WoodwardBias)
  Gen2 MCB Status/1 -> DIO - Woodward/2(Gen2 MCB Status)
  DIO - Woodward/4(Gen2 MCB) -> Gen2 MCB/1
  DIO - Woodward/2(Gen2 Fuel Enable) -> Gen2 Fuel Enable/1
  DIO - Woodward/3(Gen2 GCB) -> Gen2 GCB/1
  Woodward Primary Inputs - Gen2/1(Gen2 Gov and AVR) -> Gen2 Gov and AVR/1
  DIO - Gr3/1(DIn) -> DIO - Woodward/1(Din_Wood), Bus Creator1/1  "DIN"
  DIO - Woodward/1(DIn1) -> DIO - Gr3/1(Dout)
  Bus Creator1/1 -> Digital Inputs/1

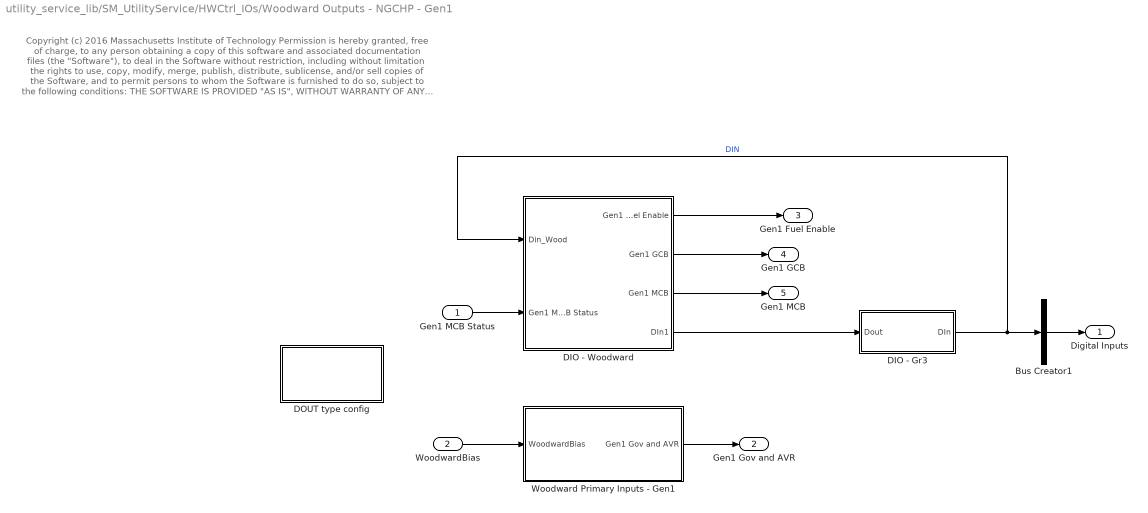
== system utility_service_lib/SM_UtilityService/HWCtrl_IOs/Woodward Outputs - NGCHP - Gen1 ==
  note: Copyright (c) 2016 Massachusetts Institute of Technology
      | Permission is hereby granted, free of charge, to any person obtaining a copy of this software and associated documentation files (the "Software"), to deal
      | in the Software without restriction, including without limitation the rights to use, copy, modify, merge, publish, distribute, sublicense, and/or sell copies of the
      | Software, and to permit persons to whom the Software is furnished to do so, subject to the following conditions:
      |
      | THE SOFTWARE IS PROVIDED "AS IS", WITHOUT WARRANTY OF ANY KIND, EXPRESS OR IMPLIED, INCLUDING BUT NOT LIMITED TO THE
      | WARRANTIES OF MERCHANTABILITY, FITNESS FOR A PARTICULAR PURPOSE AND NONINFRINGEMENT. IN NO EVENT SHALL THE AUTHORS
      | OR COPYRIGHT HOLDERS BE LIABLE FOR ANY CLAIM, DAMAGES OR OTHER LIABILITY, WHETHER IN AN ACTION OF CONTRACT, TORT OR
      | OTHERWISE, ARISING FROM, OUT OF OR IN CONNECTION WITH THE SOFTWARE OR THE USE OR OTHER DEALINGS IN THE SOFTWARE
  Gen1 MCB Status : Inport
  WoodwardBias : Inport  Port=2
  Bus Creator1 : BusCreator  Inputs=1
  DIO - Gr3 : Subsystem
  DIO - Woodward : Subsystem
  DOUT type config : Subsystem
  Woodward Primary Inputs - Gen1 : Subsystem
  Digital Inputs : Outport
  Gen1 Gov and AVR : Outport  Port=2
  Gen1 Fuel Enable : Outport  Port=3
  Gen1 GCB : Outport  Port=4
  Gen1 MCB : Outport  Port=5
  wires:
  Gen1 MCB Status/1 -> DIO - Woodward/2(Gen1 MCB Status)
  DIO - Woodward/1(Gen1 Fuel Enable) -> Gen1 Fuel Enable/1
  DIO - Woodward/3(Gen1 MCB) -> Gen1 MCB/1
  DIO - Woodward/2(Gen1 GCB) -> Gen1 GCB/1
  WoodwardBias/1 -> Woodward Primary Inputs - Gen1/1(WoodwardBias)
  Woodward Primary Inputs - Gen1/1(Gen1 Gov and AVR) -> Gen1 Gov and AVR/1
  Bus Creator1/1 -> Digital Inputs/1
  DIO - Gr3/1(DIn) -> Bus Creator1/1, DIO - Woodward/1(Din_Wood)  "DIN"
  DIO - Woodward/4(DIn1) -> DIO - Gr3/1(Dout)

== system utility_service_lib/SM_UtilityService/HWCtrl_IOs/Woodward Outputs - Diesel - Gen2/DIO - Gr3 ==
  Dout : Inport
  Bus Creator : BusCreator  Inputs=1
  Bus Selector1 : BusSelector  OutputSignals=DI_CH08-15  OutputAsBus=on
  Conditioning1 : Subsystem
  DigitalIn1 : rtio_opalrt_common/DigitalIn  CtrlName='OpCtrl'  portNb=6  FcnNos=Slot 3 Module A Subsection 2  size=1  maxcount=8  count=8  sampleTime=0  numchan=8
      settings: AttributesFormatString=%<CtrlName>
  DigitalOut1 : rtio_opalrt_common/DigitalOut  CtrlName='OpCtrl'  portNb=6  FcnNos=Slot 3 Module B Subsection 2  size=1  maxcount=8  count=8  numchan=8
      settings: AttributesFormatString=%<CtrlName>
  Terminator1 : Terminator
  Terminator6 : Terminator
  DIn : Outport
  wires:
  Conditioning1/1(Out1) -> Bus Creator/1
  Bus Creator/1 -> DIn/1
  DigitalIn1/1 -> Conditioning1/1(In1)  "DI_CH08-15"
  DigitalIn1/2 -> Terminator6/1
  Bus Selector1/1 -> DigitalOut1/1
  Dout/1 -> Bus Selector1/1
  DigitalOut1/1 -> Terminator1/1

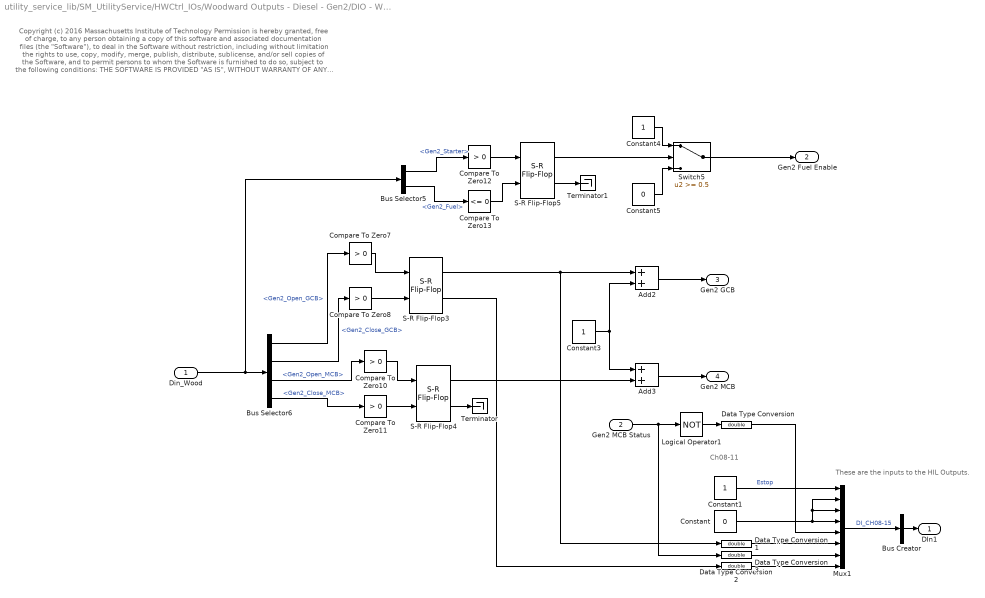
== system utility_service_lib/SM_UtilityService/HWCtrl_IOs/Woodward Outputs - Diesel - Gen2/DIO - Woodward ==
  note: These are the inputs to
      | the HIL Outputs.
  note: Ch08-11
  note: Copyright (c) 2016 Massachusetts Institute of Technology
      | Permission is hereby granted, free of charge, to any person obtaining a copy of this software and associated documentation files (the "Software"), to deal
      | in the Software without restriction, including without limitation the rights to use, copy, modify, merge, publish, distribute, sublicense, and/or sell copies of the
      | Software, and to permit persons to whom the Software is furnished to do so, subject to the following conditions:
      |
      | THE SOFTWARE IS PROVIDED "AS IS", WITHOUT WARRANTY OF ANY KIND, EXPRESS OR IMPLIED, INCLUDING BUT NOT LIMITED TO THE
      | WARRANTIES OF MERCHANTABILITY, FITNESS FOR A PARTICULAR PURPOSE AND NONINFRINGEMENT. IN NO EVENT SHALL THE AUTHORS
      | OR COPYRIGHT HOLDERS BE LIABLE FOR ANY CLAIM, DAMAGES OR OTHER LIABILITY, WHETHER IN AN ACTION OF CONTRACT, TORT OR
      | OTHERWISE, ARISING FROM, OUT OF OR IN CONNECTION WITH THE SOFTWARE OR THE USE OR OTHER DEALINGS IN THE SOFTWARE
  Din_Wood : Inport
  Gen2 MCB Status : Inport  Port=2
  Add2 : Sum
  Add3 : Sum
  Bus Creator : BusCreator  Inputs=1
  Bus Selector5 : BusSelector  OutputSignals=DI_CH08-15.Gen2_Starter,DI_CH08-15.Gen2_Fuel
  Bus Selector6 : BusSelector  OutputSignals=DI_CH08-15.Gen2_Open_GCB,DI_CH08-15.Gen2_Close_GCB,DI_CH08-15.Gen2_Open_MCB,DI_CH08-15.Gen2_Close_MCB
  Compare To Zero{7..8,10..12} (5 alike) : simulink/Logic and Bit Operations/Compare To Zero  relop=>  OutDataTypeStr=boolean
  Compare To Zero13 : simulink/Logic and Bit Operations/Compare To Zero  relop=<=  OutDataTypeStr=boolean
  Constant : Constant  Value=0
  Constant1 : Constant
  Constant3 : Constant
  Constant4 : Constant
  Constant5 : Constant  Value=0
  Data Type Conversion{,1..3} (4 alike) : DataTypeConversion  OutDataTypeStr=double
  Logical Operator1 : Logic  Operator=NOT  AllPortsSameDT=off  OutDataTypeStr=boolean
  Mux1 : Mux  Inputs=8
  S-R Flip-Flop3 : simulink_extras/Flip Flops/S-R Flip-Flop  initial_condition=1
  S-R Flip-Flop4 : simulink_extras/Flip Flops/S-R Flip-Flop  initial_condition=1
  S-R Flip-Flop5 : simulink_extras/Flip Flops/S-R Flip-Flop  initial_condition=0
  Switch5 : Switch  Threshold=0.5
  Terminator : Terminator
  Terminator1 : Terminator
  DIn1 : Outport
  Gen2 Fuel Enable : Outport  Port=2
  Gen2 GCB : Outport  Port=3
  Gen2 MCB : Outport  Port=4
  wires:
  Data Type Conversion/1 -> Mux1/5
  Logical Operator1/1 -> Data Type Conversion/1
  S-R Flip-Flop3/2 -> Data Type Conversion3/1
  Gen2 MCB Status/1 -> Data Type Conversion2/1, Logical Operator1/1
  Switch5/1 -> Gen2 Fuel Enable/1
  Compare To Zero13/1 -> S-R Flip-Flop5/2
  Constant4/1 -> Switch5/1
  Constant5/1 -> Switch5/3
  Compare To Zero12/1 -> S-R Flip-Flop5/1
  S-R Flip-Flop5/1 -> Switch5/2
  Bus Selector5/2 -> Compare To Zero13/1  "<Gen2_Fuel>"
  Bus Selector5/1 -> Compare To Zero12/1  "<Gen2_Starter>"
  Constant3/1 -> Add3/1, Add2/2
  Add3/1 -> Gen2 MCB/1
  Add2/1 -> Gen2 GCB/1
  S-R Flip-Flop4/1 -> Add3/2
  Bus Selector6/2 -> Compare To Zero8/1  "<Gen2_Close_GCB>"
  Compare To Zero10/1 -> S-R Flip-Flop4/1
  Bus Selector6/3 -> Compare To Zero10/1  "<Gen2_Open_MCB>"
  Compare To Zero11/1 -> S-R Flip-Flop4/2
  Bus Selector6/4 -> Compare To Zero11/1  "<Gen2_Close_MCB>"
  Compare To Zero8/1 -> S-R Flip-Flop3/2
  Compare To Zero7/1 -> S-R Flip-Flop3/1
  Bus Selector6/1 -> Compare To Zero7/1  "<Gen2_Open_GCB>"
  S-R Flip-Flop3/1 -> Add2/1, Data Type Conversion1/1
  Mux1/1 -> Bus Creator/1  "DI_CH08-15"
  Bus Creator/1 -> DIn1/1
  Din_Wood/1 -> Bus Selector6/1, Bus Selector5/1
  S-R Flip-Flop4/2 -> Terminator/1
  S-R Flip-Flop5/2 -> Terminator1/1
  Constant/1 -> Mux1/2, Mux1/3, Mux1/4
  Data Type Conversion1/1 -> Mux1/6
  Data Type Conversion2/1 -> Mux1/7
  Data Type Conversion3/1 -> Mux1/8
  Constant1/1 -> Mux1/1  "Estop"

== system utility_service_lib/SM_UtilityService/HWCtrl_IOs/Woodward Outputs - Diesel - Gen2/DOUT type config ==
  note: The Constants are used to select Digital Output type:
      | - 0: Time-Stamped Digital Output
      | - 1: Pulse-Width Modulated DIgital Output
  DataIn Send : rtio_opalrt_common/DataIn Send  CtrlName='OpCtrl'  FcnNos=11  width=1  portType=double  checkVersion=off  expectedId=0  expectedVersion=0  opComp=>=
      settings: AttributesFormatString=%<CtrlName>
  DataIn Send1 : rtio_opalrt_common/DataIn Send  CtrlName='OpCtrl'  FcnNos=12  width=1  portType=double  checkVersion=off  expectedId=0  expectedVersion=0  opComp=>=
      settings: AttributesFormatString=%<CtrlName>
  Subsection 3 DOUT type : Constant
  Subsection 4 DOUT type : Constant
  Terminator1 : Terminator
  Terminator2 : Terminator
  wires:
  DataIn Send/1 -> Terminator2/1
  DataIn Send1/1 -> Terminator1/1
  Subsection 4 DOUT type/1 -> DataIn Send1/1
  Subsection 3 DOUT type/1 -> DataIn Send/1

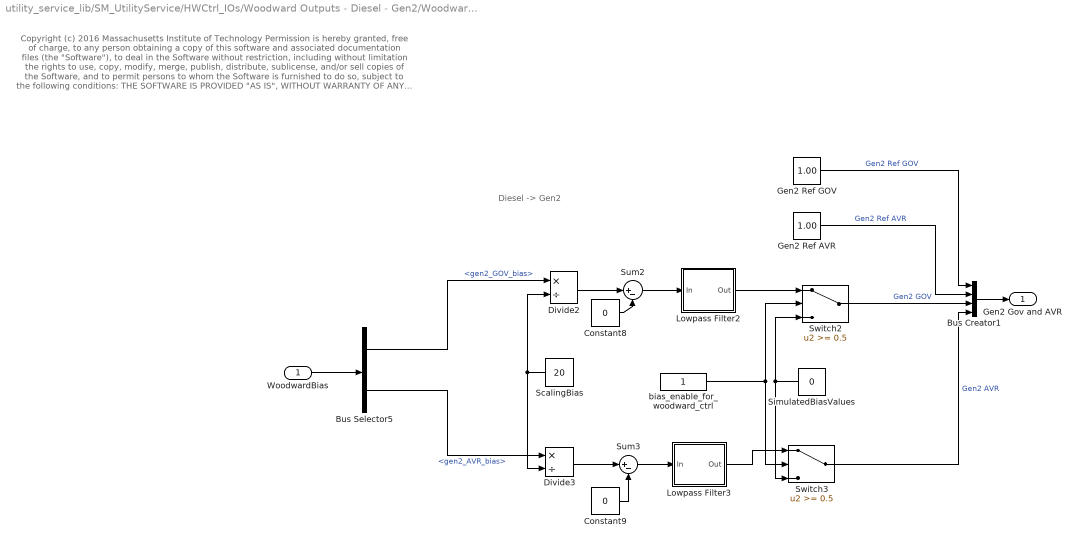
== system utility_service_lib/SM_UtilityService/HWCtrl_IOs/Woodward Outputs - Diesel - Gen2/Woodward Primary Inputs - Gen2 ==
  note: Diesel -> Gen2
  note: Copyright (c) 2016 Massachusetts Institute of Technology
      | Permission is hereby granted, free of charge, to any person obtaining a copy of this software and associated documentation files (the "Software"), to deal
      | in the Software without restriction, including without limitation the rights to use, copy, modify, merge, publish, distribute, sublicense, and/or sell copies of the
      | Software, and to permit persons to whom the Software is furnished to do so, subject to the following conditions:
      |
      | THE SOFTWARE IS PROVIDED "AS IS", WITHOUT WARRANTY OF ANY KIND, EXPRESS OR IMPLIED, INCLUDING BUT NOT LIMITED TO THE
      | WARRANTIES OF MERCHANTABILITY, FITNESS FOR A PARTICULAR PURPOSE AND NONINFRINGEMENT. IN NO EVENT SHALL THE AUTHORS
      | OR COPYRIGHT HOLDERS BE LIABLE FOR ANY CLAIM, DAMAGES OR OTHER LIABILITY, WHETHER IN AN ACTION OF CONTRACT, TORT OR
      | OTHERWISE, ARISING FROM, OUT OF OR IN CONNECTION WITH THE SOFTWARE OR THE USE OR OTHER DEALINGS IN THE SOFTWARE
  WoodwardBias : Inport
  Bus Creator1 : BusCreator
  Bus Selector5 : BusSelector  OutputSignals=gen2_GOV_bias,gen2_AVR_bias
  Constant8 : Constant  Value=0
  Constant9 : Constant  Value=0
  Divide2 : Product  Inputs=*/
  Divide3 : Product  Inputs=*/
  Gen2 Ref AVR : Constant  Value=1.00
  Gen2 Ref GOV : Constant  Value=1.00
  Lowpass Filter2 : Subsystem  DialogController=fdesignblkfcn  DialogControllerArgs=DataTag1  InitFcn=fdesignblkfcn(gcbh, {'InitFcn'});  mask(Lowpass Filter){}
      mask help: Design a lowpass filter
      settings: CopyFcn=fdesignblkfcn(gcbh, {'CopyFcn'});
      mask Help: helpview(mapfilelocation('dsp'), 'dsplowpassfilter');
      mask Display: disp('Lowpass')
  Lowpass Filter3 : Subsystem  DialogController=fdesignblkfcn  DialogControllerArgs=DataTag3  InitFcn=fdesignblkfcn(gcbh, {'InitFcn'});  mask(Lowpass Filter){}
      mask help: Design a lowpass filter
      settings: CopyFcn=fdesignblkfcn(gcbh, {'CopyFcn'});
      mask Help: helpview(mapfilelocation('dsp'), 'dsplowpassfilter');
      mask Display: disp('Lowpass')
  ScalingBias : Constant  Value=20
  SimulatedBiasValues : Constant  Value=0
  Sum2 : Sum  Inputs=|+-
  Sum3 : Sum  Inputs=|+-
  Switch2 : Switch  Threshold=0.5
  Switch3 : Switch  Threshold=0.5
  bias_enable_for_woodward_ctrl : Constant
  Gen2 Gov and AVR : Outport
  wires:
  Bus Selector5/2 -> Divide3/1  "<gen2_AVR_bias>"
  Bus Selector5/1 -> Divide2/1  "<gen2_GOV_bias>"
  WoodwardBias/1 -> Bus Selector5/1
  Bus Creator1/1 -> Gen2 Gov and AVR/1
  Gen2 Ref GOV/1 -> Bus Creator1/1  "Gen2 Ref GOV"
  Gen2 Ref AVR/1 -> Bus Creator1/2  "Gen2 Ref AVR"
  Lowpass Filter3/1(Out) -> Switch3/1
  Lowpass Filter2/1(Out) -> Switch2/1
  SimulatedBiasValues/1 -> Switch3/3, Switch2/3
  Sum3/1 -> Lowpass Filter3/1(In)
  Switch3/1 -> Bus Creator1/4  "Gen2 AVR"
  Switch2/1 -> Bus Creator1/3  "Gen2 GOV"
  Sum2/1 -> Lowpass Filter2/1(In)
  Constant9/1 -> Sum3/2
  Constant8/1 -> Sum2/2
  Divide3/1 -> Sum3/1
  Divide2/1 -> Sum2/1
  ScalingBias/1 -> Divide3/2, Divide2/2
  bias_enable_for_woodward_ctrl/1 -> Switch3/2, Switch2/2

== system utility_service_lib/SM_UtilityService/HWCtrl_IOs/Woodward Outputs - NGCHP - Gen1/DIO - Gr3 ==
  Dout : Inport
  Bus Creator : BusCreator  Inputs=1
  Bus Selector : BusSelector  OutputSignals=DI_CH00-07  OutputAsBus=on
  Conditioning : Subsystem
  DigitalIn : rtio_opalrt_common/DigitalIn  CtrlName='OpCtrl'  portNb=5  FcnNos=Slot 3 Module A Subsection 1  size=1  maxcount=8  count=8  sampleTime=0  numchan=8
      settings: AttributesFormatString=%<CtrlName>
  DigitalOut : rtio_opalrt_common/DigitalOut  CtrlName='OpCtrl'  portNb=5  FcnNos=Slot 3 Module B Subsection 1  size=1  maxcount=8  count=8  numchan=8
      settings: AttributesFormatString=%<CtrlName>
  Terminator3 : Terminator
  Terminator5 : Terminator
  DIn : Outport
  wires:
  Conditioning/1(Out1) -> Bus Creator/1
  Bus Creator/1 -> DIn/1
  DigitalIn/1 -> Conditioning/1(In1)  "DI_CH00-07"
  DigitalIn/2 -> Terminator5/1
  Bus Selector/1 -> DigitalOut/1
  Dout/1 -> Bus Selector/1
  DigitalOut/1 -> Terminator3/1

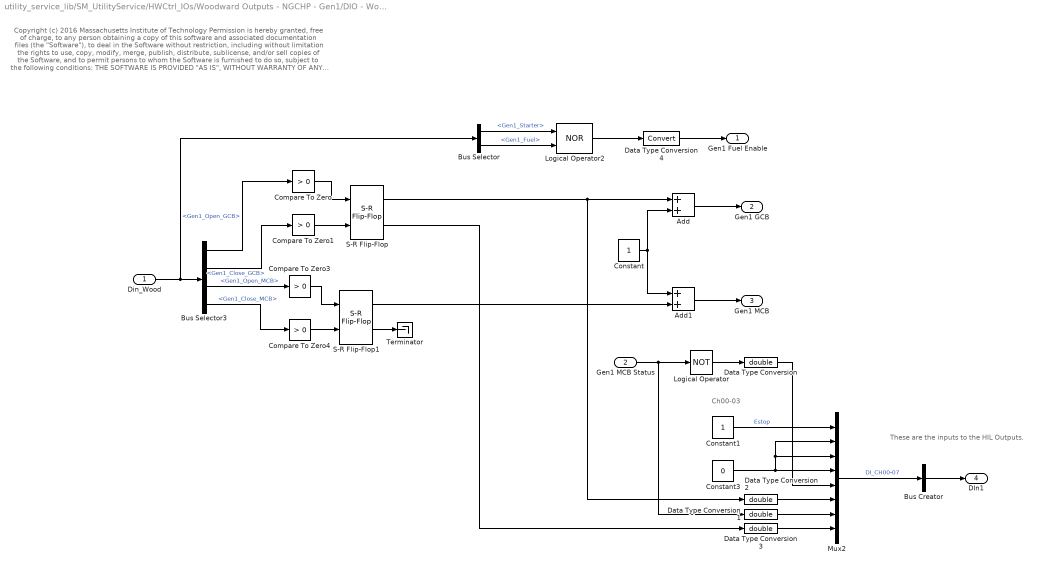
== system utility_service_lib/SM_UtilityService/HWCtrl_IOs/Woodward Outputs - NGCHP - Gen1/DIO - Woodward ==
  note: Copyright (c) 2016 Massachusetts Institute of Technology
      | Permission is hereby granted, free of charge, to any person obtaining a copy of this software and associated documentation files (the "Software"), to deal
      | in the Software without restriction, including without limitation the rights to use, copy, modify, merge, publish, distribute, sublicense, and/or sell copies of the
      | Software, and to permit persons to whom the Software is furnished to do so, subject to the following conditions:
      |
      | THE SOFTWARE IS PROVIDED "AS IS", WITHOUT WARRANTY OF ANY KIND, EXPRESS OR IMPLIED, INCLUDING BUT NOT LIMITED TO THE
      | WARRANTIES OF MERCHANTABILITY, FITNESS FOR A PARTICULAR PURPOSE AND NONINFRINGEMENT. IN NO EVENT SHALL THE AUTHORS
      | OR COPYRIGHT HOLDERS BE LIABLE FOR ANY CLAIM, DAMAGES OR OTHER LIABILITY, WHETHER IN AN ACTION OF CONTRACT, TORT OR
      | OTHERWISE, ARISING FROM, OUT OF OR IN CONNECTION WITH THE SOFTWARE OR THE USE OR OTHER DEALINGS IN THE SOFTWARE
  note: Ch00-03
  note: These are the inputs to
      | the HIL Outputs.
  Din_Wood : Inport
  Gen1 MCB Status : Inport  Port=2
  Add : Sum
  Add1 : Sum
  Bus Creator : BusCreator  Inputs=1
  Bus Selector : BusSelector  OutputSignals=DI_CH00-07.Gen1_Starter,DI_CH00-07.Gen1_Fuel
  Bus Selector3 : BusSelector  OutputSignals=DI_CH00-07.Gen1_Open_GCB,DI_CH00-07.Gen1_Close_GCB,DI_CH00-07.Gen1_Open_MCB,DI_CH00-07.Gen1_Close_MCB
  Compare To Zero{,1,3..4} (4 alike) : simulink/Logic and Bit Operations/Compare To Zero  relop=>  OutDataTypeStr=boolean
  Constant : Constant
  Constant1 : Constant
  Constant3 : Constant  Value=0
  Data Type Conversion{,1..3} (4 alike) : DataTypeConversion  OutDataTypeStr=double
  Data Type Conversion4 : DataTypeConversion
  Logical Operator : Logic  Operator=NOT  AllPortsSameDT=off  OutDataTypeStr=boolean
  Logical Operator2 : Logic  Operator=NOR  AllPortsSameDT=off  OutDataTypeStr=boolean
  Mux2 : Mux  Inputs=8
  S-R Flip-Flop : simulink_extras/Flip Flops/S-R Flip-Flop  initial_condition=1
  S-R Flip-Flop1 : simulink_extras/Flip Flops/S-R Flip-Flop  initial_condition=1
  Terminator : Terminator
  Gen1 Fuel Enable : Outport
  Gen1 GCB : Outport  Port=2
  Gen1 MCB : Outport  Port=3
  DIn1 : Outport  Port=4
  wires:
  S-R Flip-Flop1/2 -> Terminator/1
  Data Type Conversion2/1 -> Mux2/6
  Data Type Conversion1/1 -> Mux2/7
  Data Type Conversion3/1 -> Mux2/8
  Mux2/1 -> Bus Creator/1  "DI_CH00-07"
  Constant3/1 -> Mux2/2, Mux2/3, Mux2/4
  Logical Operator2/1 -> Data Type Conversion4/1
  Logical Operator/1 -> Data Type Conversion/1
  Data Type Conversion/1 -> Mux2/5
  S-R Flip-Flop/2 -> Data Type Conversion3/1
  Gen1 MCB Status/1 -> Logical Operator/1, Data Type Conversion1/1
  Bus Selector3/3 -> Compare To Zero3/1  "<Gen1_Open_MCB>"
  Bus Selector/2 -> Logical Operator2/2  "<Gen1_Fuel>"
  Bus Selector/1 -> Logical Operator2/1  "<Gen1_Starter>"
  Constant/1 -> Add1/1, Add/2
  Add1/1 -> Gen1 MCB/1
  Add/1 -> Gen1 GCB/1
  S-R Flip-Flop1/1 -> Add1/2
  Compare To Zero3/1 -> S-R Flip-Flop1/1
  Compare To Zero4/1 -> S-R Flip-Flop1/2
  Bus Selector3/4 -> Compare To Zero4/1  "<Gen1_Close_MCB>"
  Compare To Zero1/1 -> S-R Flip-Flop/2
  Compare To Zero/1 -> S-R Flip-Flop/1
  S-R Flip-Flop/1 -> Data Type Conversion2/1, Add/1
  Bus Creator/1 -> DIn1/1
  Din_Wood/1 -> Bus Selector/1, Bus Selector3/1
  Bus Selector3/1 -> Compare To Zero/1  "<Gen1_Open_GCB>"
  Bus Selector3/2 -> Compare To Zero1/1  "<Gen1_Close_GCB>"
  Data Type Conversion4/1 -> Gen1 Fuel Enable/1
  Constant1/1 -> Mux2/1  "Estop"

== system utility_service_lib/SM_UtilityService/HWCtrl_IOs/Woodward Outputs - NGCHP - Gen1/DOUT type config ==
  note: The Constants are used to select Digital Output type:
      | - 0: Time-Stamped Digital Output
      | - 1: Pulse-Width Modulated DIgital Output
  DataIn Send : rtio_opalrt_common/DataIn Send  CtrlName='OpCtrl'  FcnNos=11  width=1  portType=double  checkVersion=off  expectedId=0  expectedVersion=0  opComp=>=
      settings: AttributesFormatString=%<CtrlName>
  DataIn Send1 : rtio_opalrt_common/DataIn Send  CtrlName='OpCtrl'  FcnNos=12  width=1  portType=double  checkVersion=off  expectedId=0  expectedVersion=0  opComp=>=
      settings: AttributesFormatString=%<CtrlName>
  Subsection 3 DOUT type : Constant
  Subsection 4 DOUT type : Constant
  Terminator1 : Terminator
  Terminator2 : Terminator
  wires:
  DataIn Send/1 -> Terminator2/1
  DataIn Send1/1 -> Terminator1/1
  Subsection 4 DOUT type/1 -> DataIn Send1/1
  Subsection 3 DOUT type/1 -> DataIn Send/1

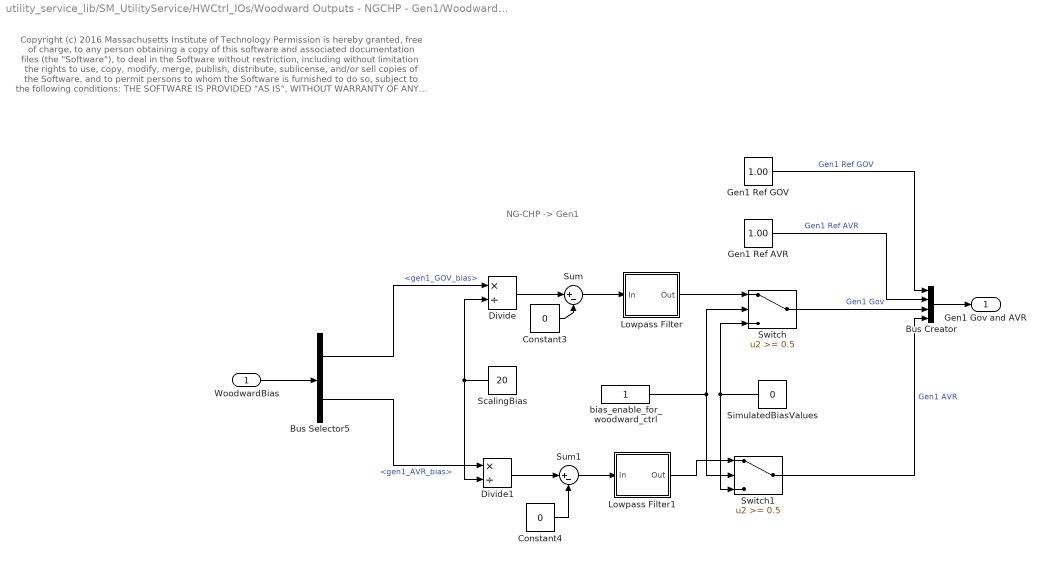
== system utility_service_lib/SM_UtilityService/HWCtrl_IOs/Woodward Outputs - NGCHP - Gen1/Woodward Primary Inputs - Gen1 ==
  note: Copyright (c) 2016 Massachusetts Institute of Technology
      | Permission is hereby granted, free of charge, to any person obtaining a copy of this software and associated documentation files (the "Software"), to deal
      | in the Software without restriction, including without limitation the rights to use, copy, modify, merge, publish, distribute, sublicense, and/or sell copies of the
      | Software, and to permit persons to whom the Software is furnished to do so, subject to the following conditions:
      |
      | THE SOFTWARE IS PROVIDED "AS IS", WITHOUT WARRANTY OF ANY KIND, EXPRESS OR IMPLIED, INCLUDING BUT NOT LIMITED TO THE
      | WARRANTIES OF MERCHANTABILITY, FITNESS FOR A PARTICULAR PURPOSE AND NONINFRINGEMENT. IN NO EVENT SHALL THE AUTHORS
      | OR COPYRIGHT HOLDERS BE LIABLE FOR ANY CLAIM, DAMAGES OR OTHER LIABILITY, WHETHER IN AN ACTION OF CONTRACT, TORT OR
      | OTHERWISE, ARISING FROM, OUT OF OR IN CONNECTION WITH THE SOFTWARE OR THE USE OR OTHER DEALINGS IN THE SOFTWARE
  note: NG-CHP -> Gen1
  WoodwardBias : Inport
  Bus Creator : BusCreator
  Bus Selector5 : BusSelector  OutputSignals=gen1_GOV_bias,gen1_AVR_bias
  Constant3 : Constant  Value=0
  Constant4 : Constant  Value=0
  Divide : Product  Inputs=*/
  Divide1 : Product  Inputs=*/
  Gen1 Ref AVR : Constant  Value=1.00
  Gen1 Ref GOV : Constant  Value=1.00
  Lowpass Filter : Subsystem  DialogController=fdesignblkfcn  DialogControllerArgs=DataTag5  InitFcn=fdesignblkfcn(gcbh, {'InitFcn'});  mask(Lowpass Filter){}
      mask help: Design a lowpass filter
      settings: CopyFcn=fdesignblkfcn(gcbh, {'CopyFcn'});
      mask Help: helpview(mapfilelocation('dsp'), 'dsplowpassfilter');
      mask Display: disp('Lowpass')
  Lowpass Filter1 : Subsystem  DialogController=fdesignblkfcn  DialogControllerArgs=DataTag7  InitFcn=fdesignblkfcn(gcbh, {'InitFcn'});  mask(Lowpass Filter){}
      mask help: Design a lowpass filter
      settings: CopyFcn=fdesignblkfcn(gcbh, {'CopyFcn'});
      mask Help: helpview(mapfilelocation('dsp'), 'dsplowpassfilter');
      mask Display: disp('Lowpass')
  ScalingBias : Constant  Value=20
  SimulatedBiasValues : Constant  Value=0
  Sum : Sum  Inputs=|+-
  Sum1 : Sum  Inputs=|+-
  Switch : Switch  Threshold=0.5
  Switch1 : Switch  Threshold=0.5
  bias_enable_for_woodward_ctrl : Constant
  Gen1 Gov and AVR : Outport
  wires:
  Bus Selector5/2 -> Divide1/1  "<gen1_AVR_bias>"
  Bus Selector5/1 -> Divide/1  "<gen1_GOV_bias>"
  WoodwardBias/1 -> Bus Selector5/1
  Bus Creator/1 -> Gen1 Gov and AVR/1
  Gen1 Ref GOV/1 -> Bus Creator/1  "Gen1 Ref GOV"
  Gen1 Ref AVR/1 -> Bus Creator/2  "Gen1 Ref AVR"
  Lowpass Filter1/1(Out) -> Switch1/1
  Lowpass Filter/1(Out) -> Switch/1
  bias_enable_for_woodward_ctrl/1 -> Switch/2, Switch1/2
  SimulatedBiasValues/1 -> Switch1/3, Switch/3
  Sum1/1 -> Lowpass Filter1/1(In)
  Switch1/1 -> Bus Creator/4  "Gen1 AVR"
  Switch/1 -> Bus Creator/3  "Gen1 Gov"
  Sum/1 -> Lowpass Filter/1(In)
  Constant4/1 -> Sum1/2
  Constant3/1 -> Sum/2
  Divide1/1 -> Sum1/1
  Divide/1 -> Sum/1
  ScalingBias/1 -> Divide1/2, Divide/2

== system utility_service_lib/SM_UtilityService/HWCtrl_IOs/Woodward Outputs - Diesel - Gen2/DIO - Gr3/Conditioning1 ==
  In1 : Inport
  Bus Creator : BusCreator  Inputs=8
  Demux : Demux  Outputs=8
  Out1 : Outport
  wires:
  Demux/1 -> Bus Creator/1  "Gen2_Starter"
  Demux/2 -> Bus Creator/2  "Gen2_Fuel"
  Demux/3 -> Bus Creator/3  "Gen2_Close_GCB"
  Demux/4 -> Bus Creator/4  "Gen2_Open_GCB"
  Demux/5 -> Bus Creator/5  "Gen2_Close_MCB"
  Demux/6 -> Bus Creator/6  "Gen2_Open_MCB"
  Demux/7 -> Bus Creator/7  "Gen2_Alarm_AB"
  Demux/8 -> Bus Creator/8  "Gen2_Alarm_CF"
  Bus Creator/1 -> Out1/1  "DI_CH08-15"
  In1/1 -> Demux/1

== system utility_service_lib/SM_UtilityService/HWCtrl_IOs/Woodward Outputs - Diesel - Gen2/Woodward Primary Inputs - Gen2/Lowpass Filter2 ==
  In : Inport
  Generated Filter Block : DiscreteFir  Tag=BlockMethodSubSystem  Coefficients=[0.0069552863617617106 0.014587901014631248 -0.0057896483056441538 -0.056861876528372622 -0.059476680260783142 0.076118200884714562 0.29579154768342669 0.40638624201187618 0.29579154768342669 0.076118200884714562 -0.059476680260783142 -0.056861876528372622 -0.0057896483056441538 0.014587901014631248 0.0069552863617617106]  InputProcessing=Columns as channels (frame based)
  Out : Outport
  wires:
  Generated Filter Block/1 -> Out/1
  In/1 -> Generated Filter Block/1

== system utility_service_lib/SM_UtilityService/HWCtrl_IOs/Woodward Outputs - Diesel - Gen2/Woodward Primary Inputs - Gen2/Lowpass Filter3 ==
  In : Inport
  Generated Filter Block : DiscreteFir  Tag=BlockMethodSubSystem  Coefficients=[0.0069552863617617106 0.014587901014631248 -0.0057896483056441538 -0.056861876528372622 -0.059476680260783142 0.076118200884714562 0.29579154768342669 0.40638624201187618 0.29579154768342669 0.076118200884714562 -0.059476680260783142 -0.056861876528372622 -0.0057896483056441538 0.014587901014631248 0.0069552863617617106]  InputProcessing=Columns as channels (frame based)
  Out : Outport
  wires:
  Generated Filter Block/1 -> Out/1
  In/1 -> Generated Filter Block/1
